simulink model "ControlSystemExercise1"  (R2019b)
settings: Solver=VariableStepAuto  StartTime=0.0  StopTime=15.0  RelTol=1e-5  AbsTol=1e-6
libraries: simulink x2
settings Model: Creator=19398  LastModifiedBy=19398

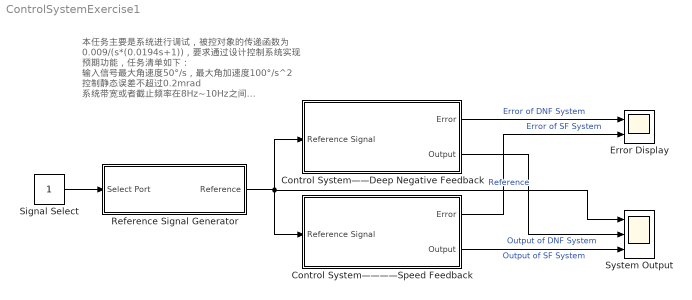
== system ControlSystemExercise1 ==
  note: 本任务主要是系统进行调试，被控对象的传递函数为
      | 0.009/(s*(0.0194s+1))，要求通过设计控制系统实现
      | 预期功能，任务清单如下：
      | 输入信号最大角速度50°/s，最大角加速度100°/s^2
      | 控制静态误差不超过0.2mrad
      | 系统带宽或者截止频率在8Hz~10Hz之间
      | 系统相角裕度大于50°
  Control System——Deep Negative Feedback : Subsystem
  Control System————Speed Feedback : Subsystem
  Error Display : Scope  NumInputPorts=2
  Reference Signal Generator : Subsystem
  Signal Select : Constant
  System Output : Scope  NumInputPorts=3
  wires:
  Reference Signal Generator/1(Reference) -> Control System————Speed Feedback/1(Reference Signal), System Output/1, Control System——Deep Negative Feedback/1(Reference Signal)  "Reference"
  Signal Select/1 -> Reference Signal Generator/1(Select Port)
  Control System——Deep Negative Feedback/1(Error) -> Error Display/1  "Error of DNF System"
  Control System————Speed Feedback/1(Error) -> Error Display/2  "Error of SF System"
  Control System——Deep Negative Feedback/2(Output) -> System Output/2  "Output of DNF System"
  Control System————Speed Feedback/2(Output) -> System Output/3  "Output of SF System"

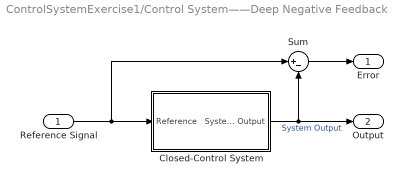
== system ControlSystemExercise1/Control System——Deep Negative Feedback ==
  Reference Signal : Inport
  Closed-Control System : Subsystem
  Sum : Sum  Inputs=|+-
  Error : Outport
  Output : Outport  Port=2
  wires:
  Sum/1 -> Error/1
  Reference Signal/1 -> Sum/1, Closed-Control System/1(Reference)
  Closed-Control System/1(System Output) -> Output/1, Sum/2  "System Output"

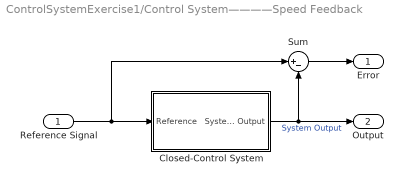
== system ControlSystemExercise1/Control System————Speed Feedback ==
  Reference Signal : Inport
  Closed-Control System : Subsystem
  Sum : Sum  Inputs=|+-
  Error : Outport
  Output : Outport  Port=2
  wires:
  Sum/1 -> Error/1
  Reference Signal/1 -> Sum/1, Closed-Control System/1(Reference)
  Closed-Control System/1(System Output) -> Output/1, Sum/2  "System Output"

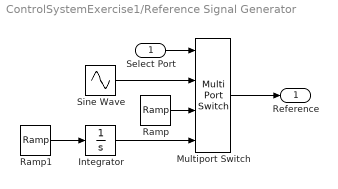
== system ControlSystemExercise1/Reference Signal Generator ==
  Select Port : Inport
  Integrator : Integrator
  Multiport Switch : MultiPortSwitch
  Ramp : simulink/Sources/Ramp  slope=50  start=0  InitialOutput=0
  Ramp1 : simulink/Sources/Ramp  slope=100  start=0  InitialOutput=0
  Sine Wave : Sin  Amplitude=50  Frequency=2  SampleTime=0
  Reference : Outport
  wires:
  Select Port/1 -> Multiport Switch/1
  Multiport Switch/1 -> Reference/1
  Sine Wave/1 -> Multiport Switch/2
  Ramp/1 -> Multiport Switch/3
  Ramp1/1 -> Integrator/1
  Integrator/1 -> Multiport Switch/4

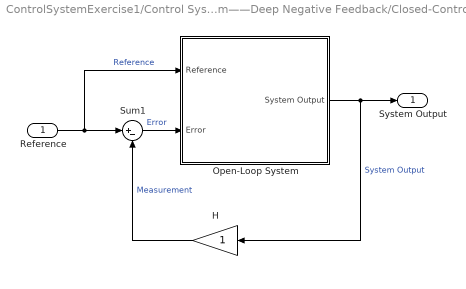
== system ControlSystemExercise1/Control System——Deep Negative Feedback/Closed-Control System ==
  Reference : Inport
  H : Gain
  Open-Loop System : Subsystem
  Sum1 : Sum  Inputs=|+-
  System Output : Outport
  wires:
  Reference/1 -> Open-Loop System/1(Reference), Sum1/1  "Reference"
  H/1 -> Sum1/2  "Measurement"
  Open-Loop System/1(System Output) -> System Output/1, H/1  "System Output"
  Sum1/1 -> Open-Loop System/2(Error)  "Error"

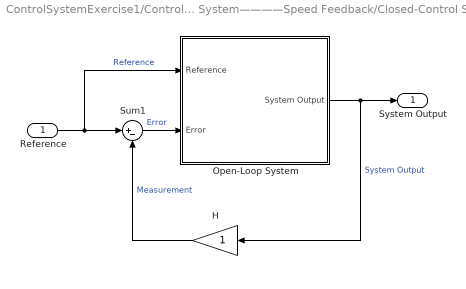
== system ControlSystemExercise1/Control System————Speed Feedback/Closed-Control System ==
  Reference : Inport
  H : Gain
  Open-Loop System : Subsystem
  Sum1 : Sum  Inputs=|+-
  System Output : Outport
  wires:
  Reference/1 -> Open-Loop System/1(Reference), Sum1/1  "Reference"
  H/1 -> Sum1/2  "Measurement"
  Open-Loop System/1(System Output) -> System Output/1, H/1  "System Output"
  Sum1/1 -> Open-Loop System/2(Error)  "Error"

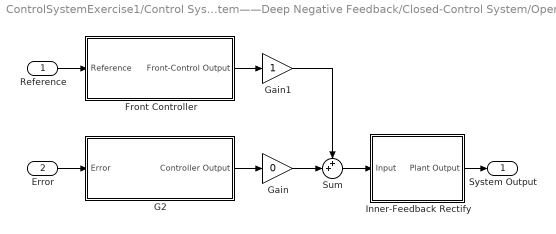
== system ControlSystemExercise1/Control System——Deep Negative Feedback/Closed-Control System/Open-Loop System ==
  Reference : Inport
  Error : Inport  Port=2
  Front Controller : Subsystem
  G2 : Subsystem
  Gain : Gain  Gain=0
  Gain1 : Gain
  Inner-Feedback Rectify : Subsystem
  Sum : Sum  Inputs=++|
  System Output : Outport
  wires:
  Sum/1 -> Inner-Feedback Rectify/1(Input)
  Gain/1 -> Sum/2
  Reference/1 -> Front Controller/1(Reference)
  Inner-Feedback Rectify/1(Plant Output) -> System Output/1
  Error/1 -> G2/1(Error)
  G2/1(Controller Output) -> Gain/1
  Gain1/1 -> Sum/1
  Front Controller/1(Front-Control Output) -> Gain1/1

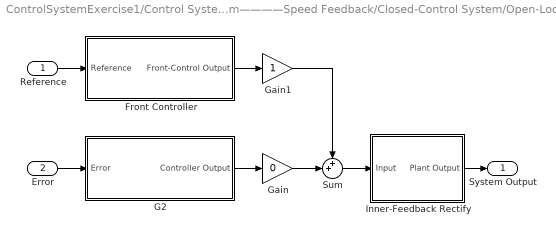
== system ControlSystemExercise1/Control System————Speed Feedback/Closed-Control System/Open-Loop System ==
  Reference : Inport
  Error : Inport  Port=2
  Front Controller : Subsystem
  G2 : Subsystem
  Gain : Gain  Gain=0
  Gain1 : Gain
  Inner-Feedback Rectify : Subsystem
  Sum : Sum  Inputs=++|
  System Output : Outport
  wires:
  Sum/1 -> Inner-Feedback Rectify/1(Input)
  Gain/1 -> Sum/2
  Reference/1 -> Front Controller/1(Reference)
  Inner-Feedback Rectify/1(Plant Output) -> System Output/1
  Error/1 -> G2/1(Error)
  G2/1(Controller Output) -> Gain/1
  Gain1/1 -> Sum/1
  Front Controller/1(Front-Control Output) -> Gain1/1

== system ControlSystemExercise1/Control System——Deep Negative Feedback/Closed-Control System/Open-Loop System/Front Controller ==
  Reference : Inport
  G3 : Gain  Gain=300
  Transfer Fcn : TransferFcn  Denominator=[0.002 1]
  Front-Control Output : Outport
  wires:
  Reference/1 -> G3/1
  G3/1 -> Transfer Fcn/1
  Transfer Fcn/1 -> Front-Control Output/1

== system ControlSystemExercise1/Control System——Deep Negative Feedback/Closed-Control System/Open-Loop System/G2 ==
  Error : Inport
  Gain1 : Gain  Gain=23000
  Transfer Fcn : TransferFcn  Numerator=[0.0265 1]  Denominator="[0.0003    0.0398    1.0000 0]"
  Controller Output : Outport
  wires:
  Error/1 -> Gain1/1
  Gain1/1 -> Transfer Fcn/1
  Transfer Fcn/1 -> Controller Output/1

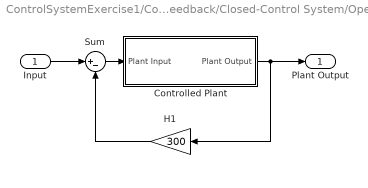
== system ControlSystemExercise1/Control System——Deep Negative Feedback/Closed-Control System/Open-Loop System/Inner-Feedback Rectify ==
  Input : Inport
  Controlled Plant : Subsystem
  H1 : Gain  Gain=300
  Sum : Sum  Inputs=|+-
  Plant Output : Outport
  wires:
  Controlled Plant/1(Plant Output) -> H1/1, Plant Output/1
  H1/1 -> Sum/2
  Sum/1 -> Controlled Plant/1(Plant Input)
  Input/1 -> Sum/1

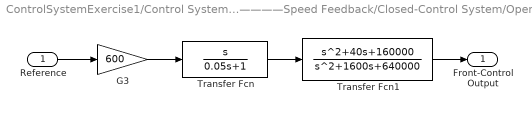
== system ControlSystemExercise1/Control System————Speed Feedback/Closed-Control System/Open-Loop System/Front Controller ==
  Reference : Inport
  G3 : Gain  Gain=600
  Transfer Fcn : TransferFcn  Numerator=[1 0]  Denominator=[0.05 1]
  Transfer Fcn1 : TransferFcn  Numerator=[1 40 160000]  Denominator=[1 1600 640000]
  Front-Control Output : Outport
  wires:
  Reference/1 -> G3/1
  G3/1 -> Transfer Fcn/1
  Transfer Fcn/1 -> Transfer Fcn1/1
  Transfer Fcn1/1 -> Front-Control Output/1

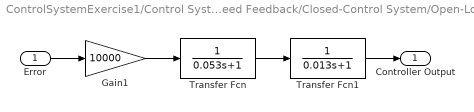
== system ControlSystemExercise1/Control System————Speed Feedback/Closed-Control System/Open-Loop System/G2 ==
  Error : Inport
  Gain1 : Gain  Gain=10000
  Transfer Fcn : TransferFcn  Denominator=[0.053 1]
  Transfer Fcn1 : TransferFcn  Denominator=[0.013 1]
  Controller Output : Outport
  wires:
  Error/1 -> Gain1/1
  Gain1/1 -> Transfer Fcn/1
  Transfer Fcn/1 -> Transfer Fcn1/1
  Transfer Fcn1/1 -> Controller Output/1

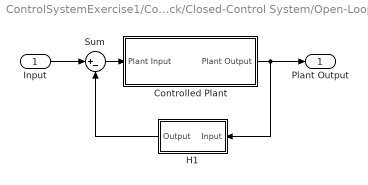
== system ControlSystemExercise1/Control System————Speed Feedback/Closed-Control System/Open-Loop System/Inner-Feedback Rectify ==
  Input : Inport
  Controlled Plant : Subsystem
  H1 : Subsystem
  Sum : Sum  Inputs=|+-
  Plant Output : Outport
  wires:
  Controlled Plant/1(Plant Output) -> H1/1(Input), Plant Output/1
  Sum/1 -> Controlled Plant/1(Plant Input)
  Input/1 -> Sum/1
  H1/1(Output) -> Sum/2

== system ControlSystemExercise1/Control System——Deep Negative Feedback/Closed-Control System/Open-Loop System/Inner-Feedback Rectify/Controlled Plant ==
  Plant Input : Inport
  G2 : Subsystem
  Plant : Subsystem
  Plant Output : Outport
  wires:
  Plant/1(System Output) -> Plant Output/1
  Plant Input/1 -> G2/1(Input)
  G2/1(Output) -> Plant/1(Controlled Variable)

== system ControlSystemExercise1/Control System————Speed Feedback/Closed-Control System/Open-Loop System/Inner-Feedback Rectify/Controlled Plant ==
  Plant Input : Inport
  G2 : Subsystem
  Plant : Subsystem
  Plant Output : Outport
  wires:
  Plant/1(System Output) -> Plant Output/1
  Plant Input/1 -> G2/1(Input)
  G2/1(Output) -> Plant/1(Controlled Variable)

== system ControlSystemExercise1/Control System————Speed Feedback/Closed-Control System/Open-Loop System/Inner-Feedback Rectify/H1 ==
  Input : Inport
  Derivative : Derivative  CoefficientInTFapproximation=0.05
  Gain : Gain  Gain=150
  Output : Outport
  wires:
  Gain/1 -> Output/1
  Input/1 -> Derivative/1
  Derivative/1 -> Gain/1

== system ControlSystemExercise1/Control System——Deep Negative Feedback/Closed-Control System/Open-Loop System/Inner-Feedback Rectify/Controlled Plant/G2 ==
  Input : Inport
  Transfer Fcn : TransferFcn  Numerator=[0.02 1]  Denominator=[0.002 1]
  gain : Gain  Gain=400
  Output : Outport
  wires:
  gain/1 -> Transfer Fcn/1
  Input/1 -> gain/1
  Transfer Fcn/1 -> Output/1

== system ControlSystemExercise1/Control System——Deep Negative Feedback/Closed-Control System/Open-Loop System/Inner-Feedback Rectify/Controlled Plant/Plant ==
  Controlled Variable : Inport
  Gain : Gain  Gain=0.5
  Object : TransferFcn  Numerator=[0.018]  Denominator=[0.0194 1 0]
  System Output : Outport
  wires:
  Object/1 -> Gain/1
  Controlled Variable/1 -> Object/1
  Gain/1 -> System Output/1

== system ControlSystemExercise1/Control System————Speed Feedback/Closed-Control System/Open-Loop System/Inner-Feedback Rectify/Controlled Plant/G2 ==
  Input : Inport
  gain : Gain  Gain=140
  Output : Outport
  wires:
  Input/1 -> gain/1
  gain/1 -> Output/1

== system ControlSystemExercise1/Control System————Speed Feedback/Closed-Control System/Open-Loop System/Inner-Feedback Rectify/Controlled Plant/Plant ==
  Controlled Variable : Inport
  Gain : Gain  Gain=0.5
  Object : TransferFcn  Numerator=[0.018]  Denominator=[0.0194 1 0]
  System Output : Outport
  wires:
  Object/1 -> Gain/1
  Controlled Variable/1 -> Object/1
  Gain/1 -> System Output/1
